simulink model "Master_Slave_No_Force_Control"  (R2020a)
settings: Solver=VariableStepAuto  StartTime=0.0  StopTime=1000  RelTol=1e-3
values from neighbouring files (symbols this model uses):
  B = 100    [Teleop_parameters.m]    (also in base.mat = 0.0517063081696; base_no_attrito.mat = 0; ci_siamo.mat = 0.0517063081696; force_control.mat = 0.0517063081696)
  Be = 10^3    (= 1000)    [Teleop_parameters.m]    (also in base.mat = 0.5; base_no_attrito.mat = 0.5; ci_siamo.mat = 5; force_control.mat = 0.5)
  Bh = 0.02    [Teleop_parameters.m]    (also in base.mat; base_no_attrito.mat; ci_siamo.mat; force_control.mat)
  Bl = 0.02    [Teleop_parameters.m]
  Fc_h = 5    [Teleop_parameters.m]    (also in base.mat; base_no_attrito.mat; ci_siamo.mat; force_control.mat)
  J = 50    [Teleop_parameters.m]    (also in base.mat = 0.0629265770424; base_no_attrito.mat = 0.0629265770424; ci_siamo.mat = 0.0629265770424; force_control.mat = 0.0629265770424)
  Jh = 0.02    [Teleop_parameters.m]    (also in base.mat; base_no_attrito.mat; ci_siamo.mat; force_control.mat)
  Jl = 0.03    [Teleop_parameters.m]
  Kc2v_m = 2    [Teleop_parameters.m]    (also in base.mat; base_no_attrito.mat; ci_siamo.mat; force_control.mat)
  Kc2v_s = 2    [Teleop_parameters.m]    (also in base.mat; base_no_attrito.mat; ci_siamo.mat; force_control.mat)
  Kd_h = 0.5    [Teleop_parameters.m]    (also in base.mat = 1; base_no_attrito.mat = 1; ci_siamo.mat = 10; force_control.mat = 1)
  Kd_m = 6    [Teleop_parameters.m]    (also in base.mat = 1; base_no_attrito.mat = 1; ci_siamo.mat = 0.005; force_control.mat = 1)
  Kd_s = 6    [Teleop_parameters.m]    (also in base.mat = 1; base_no_attrito.mat = 1; ci_siamo.mat = 0.5; force_control.mat = 1)
  Ke = 2    [Teleop_parameters.m]    (also in base.mat = 10; base_no_attrito.mat = 10; ci_siamo.mat = 10; force_control.mat = 10)
  Km = 2    [Teleop_parameters.m]
  Kp_h = 1.2    [Teleop_parameters.m]    (also in base.mat; base_no_attrito.mat; ci_siamo.mat = 10; force_control.mat)
  Kp_m = 200    [Teleop_parameters.m]    (also in base.mat = 1; base_no_attrito.mat = 1; ci_siamo.mat = 0.01; force_control.mat = 1)
  Kp_s = 200    [Teleop_parameters.m]    (also in base.mat = 1; base_no_attrito.mat = 1; ci_siamo.mat = 1; force_control.mat = 1)
  Kt2c_m = 1.182    [Teleop_parameters.m]    (also in base.mat; base_no_attrito.mat; ci_siamo.mat; force_control.mat)
  Kt2c_s = 1.182    [Teleop_parameters.m]    (also in base.mat; base_no_attrito.mat; ci_siamo.mat; force_control.mat)
  L = 0.0025    [Teleop_parameters.m]
  lArm_m = 0.1    [Teleop_parameters.m]    (also in base.mat; base_no_attrito.mat; ci_siamo.mat; force_control.mat)
  lArm_s = 0.1    [Teleop_parameters.m]    (also in base.mat; base_no_attrito.mat; ci_siamo.mat; force_control.mat)
  maxCurrent_m = 4.5    [Teleop_parameters.m]    (also in base.mat; base_no_attrito.mat; ci_siamo.mat; force_control.mat)
  maxCurrent_s = 4.5    [Teleop_parameters.m]    (also in base.mat; base_no_attrito.mat; ci_siamo.mat; force_control.mat)
  N = 1    [Teleop_parameters.m]
  qe = 1    [Teleop_parameters.m]    (also in base.mat = 5; base_no_attrito.mat = 5; ci_siamo.mat = 0.5; force_control.mat = 5)
  R = 0.434    [Teleop_parameters.m]
settings Model: Creator=kriato  LastModifiedBy=giovanni

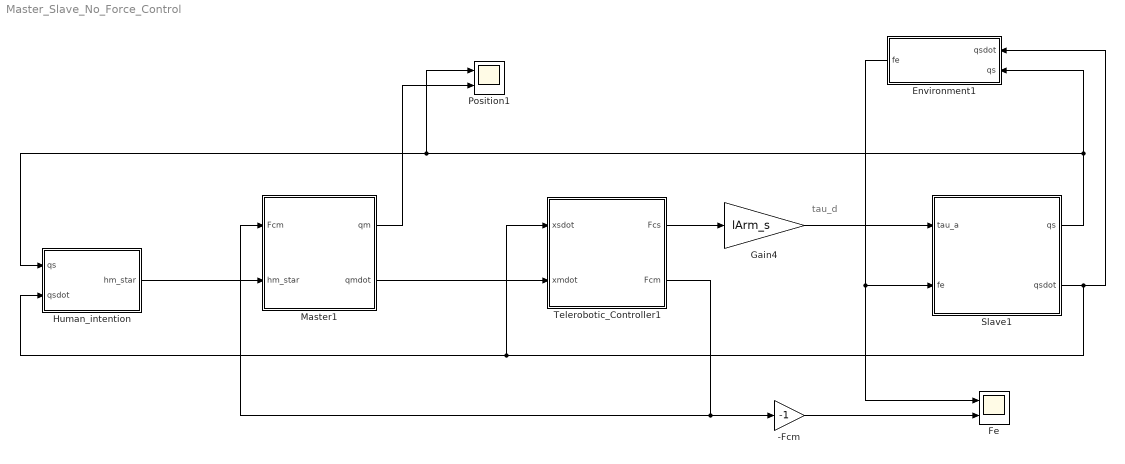
== system Master_Slave_No_Force_Control ==
  note: tau_d
  -Fcm : Gain  Gain=-1
  Environment1 : Subsystem
  Fe : Scope  NumInputPorts=2
  Gain4 : Gain  Gain=lArm_s
  Human_intention : Subsystem
  Master1 : Subsystem
  Position1 : Scope  NumInputPorts=2
  Slave1 : Subsystem
  Telerobotic_Controller1 : Subsystem
  wires:
  Gain4/1 -> Slave1/1(tau_a)
  Master1/1(qm) -> Position1/2
  Environment1/1(fe) -> Fe/1, Slave1/2(fe)
  Telerobotic_Controller1/1(Fcs) -> Gain4/1
  Slave1/1(qs) -> Environment1/2(qs), Human_intention/1(qs), Position1/1
  Telerobotic_Controller1/2(Fcm) -> Master1/1(Fcm), -Fcm/1
  -Fcm/1 -> Fe/2
  Slave1/2(qsdot) -> Human_intention/2(qsdot), Telerobotic_Controller1/1(xsdot), Environment1/1(qsdot)
  Human_intention/1(hm_star) -> Master1/2(hm_star)
  Master1/2(qmdot) -> Telerobotic_Controller1/2(xmdot)

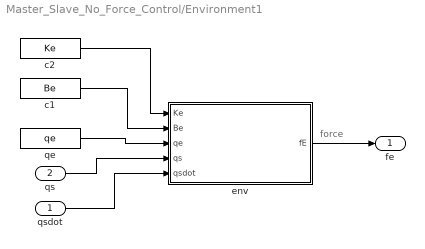
== system Master_Slave_No_Force_Control/Environment1 ==
  note: force
  qsdot : Inport
  qs : Inport  Port=2
  c1 : Constant  Value=Be  SampleTime=0
  c2 : Constant  Value=Ke  SampleTime=0
  env : MATLAB Function  TreatAsAtomicUnit=on
  qe : Constant  Value=qe  SampleTime=0
  fe : Outport  VectorParamsAs1DForOutWhenUnconnected=off
  wires:
  qe/1 -> env/3(qe)
  c1/1 -> env/2(Be)
  c2/1 -> env/1(Ke)
  qs/1 -> env/4(qs)
  qsdot/1 -> env/5(qsdot)
  env/1(fE) -> fe/1

== system Master_Slave_No_Force_Control/Human_intention ==
  qs : Inport
  qsdot : Inport  Port=2
  Operator (intention) : Subsystem
  Subsystem : Subsystem
  hm_star : Outport
  wires:
  Subsystem/1(qm_ref) -> Operator (intention)/3(qm_ref)
  Subsystem/2(qmdot_ref) -> Operator (intention)/4(qmdot_ref)
  Operator (intention)/1(hm_star) -> hm_star/1
  qs/1 -> Operator (intention)/1(qs)
  qsdot/1 -> Operator (intention)/2(qsdot)

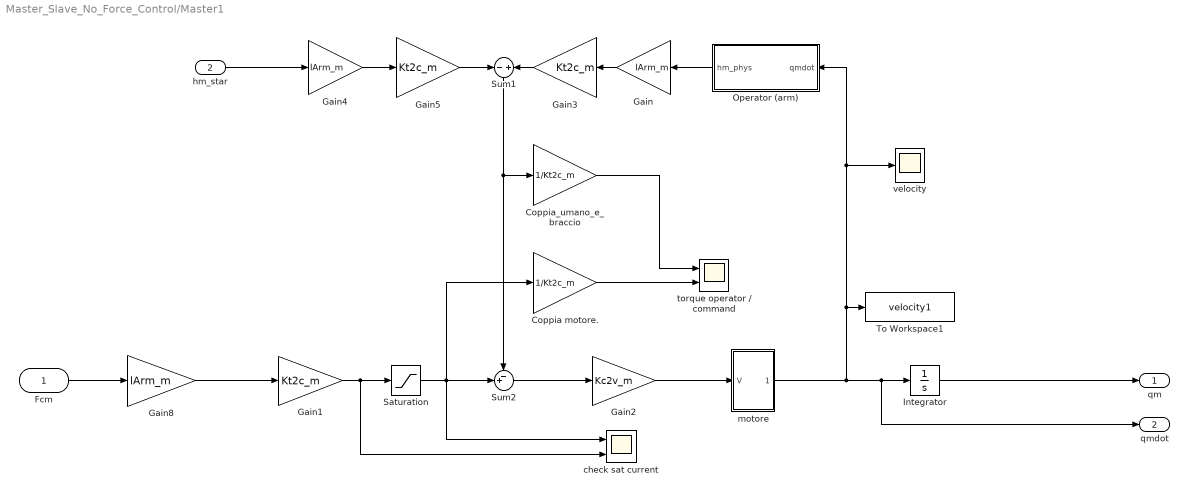
== system Master_Slave_No_Force_Control/Master1 ==
  Fcm : Inport
  hm_star : Inport  Port=2
  Coppia motore. : Gain  Gain=1/Kt2c_m
  Coppia_umano_e_braccio : Gain  Gain=1/Kt2c_m
  Gain : Gain  Gain=lArm_m
  Gain1 : Gain  Gain=Kt2c_m
  Gain2 : Gain  Gain=Kc2v_m
  Gain3 : Gain  Gain=Kt2c_m
  Gain4 : Gain  Gain=lArm_m
  Gain5 : Gain  Gain=Kt2c_m
  Gain8 : Gain  Gain=lArm_m
  Integrator : Integrator
  Operator (arm) : Subsystem
  Saturation : Saturate  UpperLimit=maxCurrent_m  LowerLimit=-maxCurrent_m
  Sum1 : Sum  Inputs=-+
  Sum2 : Sum  Inputs=-+|
  To Workspace1 : ToWorkspace  VariableName=velocity1  SaveFormat=Timeseries  SampleTime=-1
  check sat current : Scope  NumInputPorts=2
  motore : Subsystem
  torque operator / command : Scope  NumInputPorts=2
  velocity : Scope
  qm : Outport
  qmdot : Outport  Port=2
  wires:
  Integrator/1 -> qm/1
  Sum2/1 -> Gain2/1
  Gain3/1 -> Sum1/2
  Gain2/1 -> motore/1(V)
  Gain1/1 -> check sat current/2, Saturation/1
  Coppia_umano_e_braccio/1 -> torque operator / command/1
  Coppia motore./1 -> torque operator / command/2
  motore/1(qdot) -> velocity/1, Operator (arm)/1(qmdot), To Workspace1/1, qmdot/1, Integrator/1
  Gain8/1 -> Gain1/1
  Gain5/1 -> Sum1/1
  Operator (arm)/1(hm_phys) -> Gain/1
  Sum1/1 -> Sum2/1, Coppia_umano_e_braccio/1
  Saturation/1 -> Coppia motore./1, Sum2/2, check sat current/1
  Gain/1 -> Gain3/1
  Gain4/1 -> Gain5/1
  Fcm/1 -> Gain8/1
  hm_star/1 -> Gain4/1

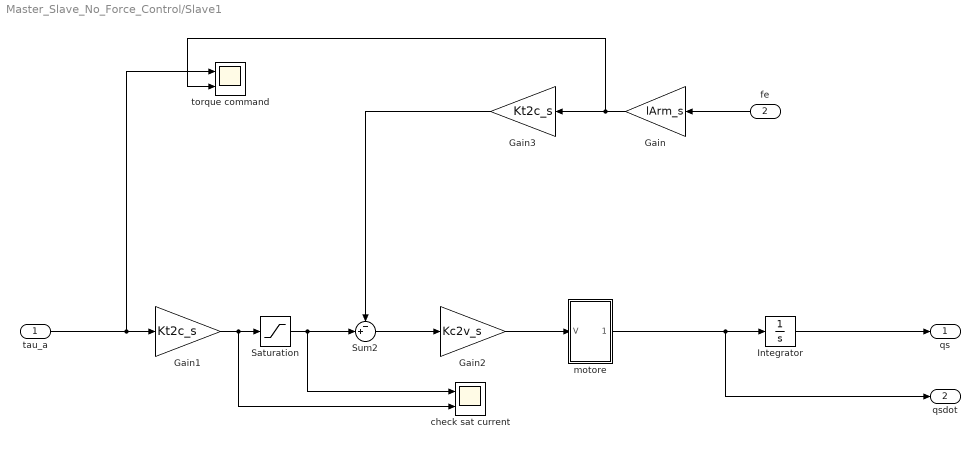
== system Master_Slave_No_Force_Control/Slave1 ==
  tau_a : Inport
  fe : Inport  Port=2
  Gain : Gain  Gain=lArm_s
  Gain1 : Gain  Gain=Kt2c_s
  Gain2 : Gain  Gain=Kc2v_s
  Gain3 : Gain  Gain=Kt2c_s
  Integrator : Integrator
  Saturation : Saturate  UpperLimit=maxCurrent_s  LowerLimit=-maxCurrent_s
  Sum2 : Sum  Inputs=-+|
  check sat current : Scope  NumInputPorts=2
  motore : Subsystem
  torque command : Scope  NumInputPorts=2
  qs : Outport
  qsdot : Outport  Port=2
  wires:
  Integrator/1 -> qs/1
  Sum2/1 -> Gain2/1
  Saturation/1 -> Sum2/2, check sat current/1
  Gain2/1 -> motore/1(V)
  motore/1(qdot) -> qsdot/1, Integrator/1
  Gain1/1 -> check sat current/2, Saturation/1
  tau_a/1 -> torque command/1, Gain1/1
  Gain3/1 -> Sum2/1
  fe/1 -> Gain/1
  Gain/1 -> Gain3/1, torque command/2

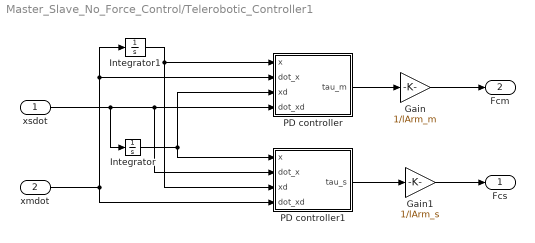
== system Master_Slave_No_Force_Control/Telerobotic_Controller1 ==
  xsdot : Inport
  xmdot : Inport  Port=2
  Gain : Gain  Gain=1/lArm_m
  Gain1 : Gain  Gain=1/lArm_s
  Integrator : Integrator
  Integrator1 : Integrator
  PD controller : Subsystem
  PD controller1 : Subsystem
  Fcs : Outport
  Fcm : Outport  Port=2
  wires:
  Integrator/1 -> PD controller1/1(x), PD controller/3(xd)
  Integrator1/1 -> PD controller1/3(xd), PD controller/1(x)
  xsdot/1 -> PD controller1/2(dot_x), PD controller/4(dot_xd), Integrator/1
  PD controller1/1(tau_s) -> Gain1/1
  PD controller/1(tau_m) -> Gain/1
  xmdot/1 -> PD controller1/4(dot_xd), PD controller/2(dot_x), Integrator1/1
  Gain/1 -> Fcm/1
  Gain1/1 -> Fcs/1

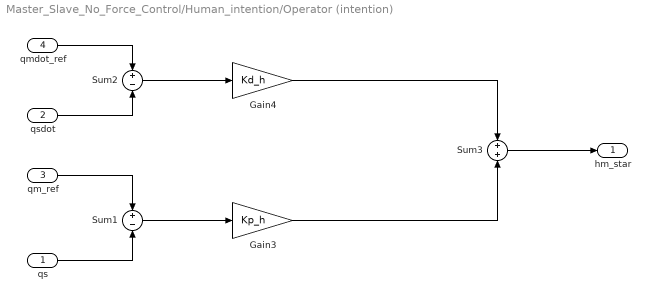
== system Master_Slave_No_Force_Control/Human_intention/Operator (intention) ==
  qs : Inport
  qsdot : Inport  Port=2
  qm_ref : Inport  Port=3
  qmdot_ref : Inport  Port=4
  Gain3 : Gain  Gain=Kp_h
  Gain4 : Gain  Gain=Kd_h
  Sum1 : Sum  Inputs=+|-
  Sum2 : Sum  Inputs=+|-
  Sum3 : Sum  Inputs=+|+
  hm_star : Outport  VectorParamsAs1DForOutWhenUnconnected=off
  wires:
  qs/1 -> Sum1/2
  qm_ref/1 -> Sum1/1
  qmdot_ref/1 -> Sum2/1
  Sum1/1 -> Gain3/1
  qsdot/1 -> Sum2/2
  Sum2/1 -> Gain4/1
  Gain4/1 -> Sum3/1
  Gain3/1 -> Sum3/2
  Sum3/1 -> hm_star/1

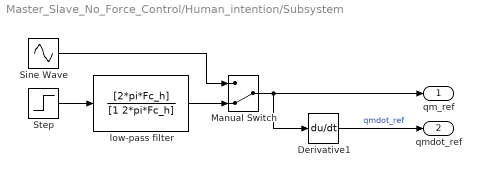
== system Master_Slave_No_Force_Control/Human_intention/Subsystem ==
  Derivative1 : Derivative  CoefficientInTFapproximation=0.001
  Manual Switch : ManualSwitch  CurrentSetting=0
  Sine Wave : Sin  SampleTime=0
  Step : Step  SampleTime=0
  low-pass filter : TransferFcn  Numerator=[2*pi*Fc_h]  Denominator=[1 2*pi*Fc_h]
  qm_ref : Outport
  qmdot_ref : Outport  Port=2
  wires:
  low-pass filter/1 -> Manual Switch/2
  Manual Switch/1 -> qm_ref/1, Derivative1/1
  Derivative1/1 -> qmdot_ref/1  "qmdot_ref"
  Step/1 -> low-pass filter/1
  Sine Wave/1 -> Manual Switch/1

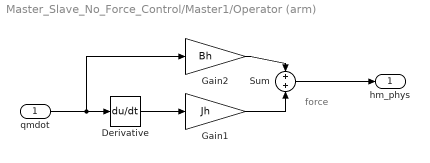
== system Master_Slave_No_Force_Control/Master1/Operator (arm) ==
  note: force
  qmdot : Inport
  Derivative : Derivative  CoefficientInTFapproximation=0.001
  Gain1 : Gain  Gain=Jh
  Gain2 : Gain  Gain=Bh
  Sum : Sum  Inputs=+|+
  hm_phys : Outport  VectorParamsAs1DForOutWhenUnconnected=off
  wires:
  qmdot/1 -> Gain2/1, Derivative/1
  Sum/1 -> hm_phys/1
  Derivative/1 -> Gain1/1
  Gain2/1 -> Sum/1
  Gain1/1 -> Sum/2

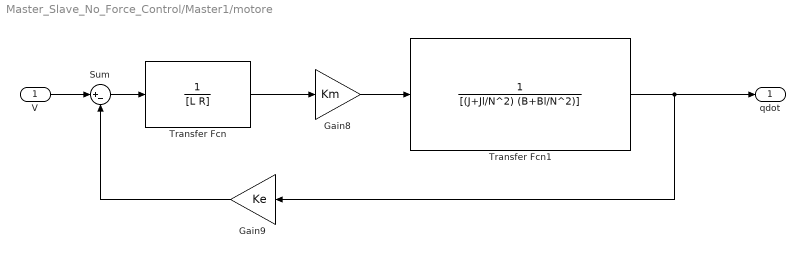
== system Master_Slave_No_Force_Control/Master1/motore ==
  V : Inport
  Gain8 : Gain  Gain=Km
  Gain9 : Gain  Gain=Ke
  Sum : Sum  Inputs=|+-
  Transfer Fcn : TransferFcn  Denominator=[L R]
  Transfer Fcn1 : TransferFcn  Denominator=[(J+Jl/N^2) (B+Bl/N^2)]
  qdot : Outport
  wires:
  Sum/1 -> Transfer Fcn/1
  V/1 -> Sum/1
  Transfer Fcn/1 -> Gain8/1
  Gain9/1 -> Sum/2
  Gain8/1 -> Transfer Fcn1/1
  Transfer Fcn1/1 -> Gain9/1, qdot/1

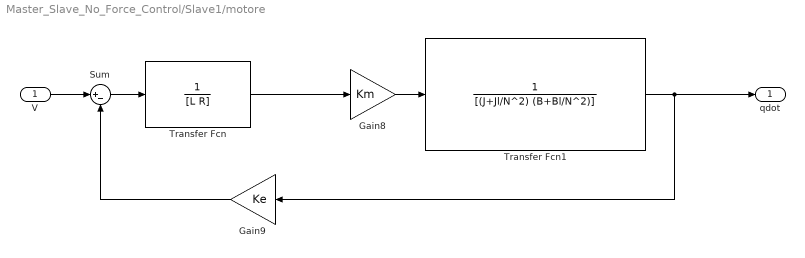
== system Master_Slave_No_Force_Control/Slave1/motore ==
  V : Inport
  Gain8 : Gain  Gain=Km
  Gain9 : Gain  Gain=Ke
  Sum : Sum  Inputs=|+-
  Transfer Fcn : TransferFcn  Denominator=[L R]
  Transfer Fcn1 : TransferFcn  Denominator=[(J+Jl/N^2) (B+Bl/N^2)]
  qdot : Outport
  wires:
  Sum/1 -> Transfer Fcn/1
  V/1 -> Sum/1
  Transfer Fcn/1 -> Gain8/1
  Gain9/1 -> Sum/2
  Gain8/1 -> Transfer Fcn1/1
  Transfer Fcn1/1 -> Gain9/1, qdot/1

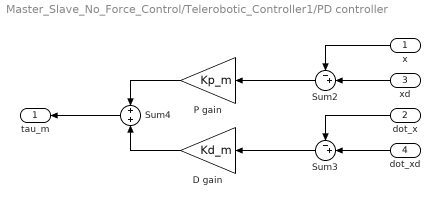
== system Master_Slave_No_Force_Control/Telerobotic_Controller1/PD controller ==
  x : Inport
  dot_x : Inport  Port=2
  xd : Inport  Port=3
  dot_xd : Inport  Port=4
  D gain : Gain  Gain=Kd_m
  P gain : Gain  Gain=Kp_m
  Sum2 : Sum  Inputs=-+|
  Sum3 : Sum  Inputs=-+|
  Sum4 : Sum
  tau_m : Outport  VectorParamsAs1DForOutWhenUnconnected=off
  wires:
  D gain/1 -> Sum4/2
  dot_x/1 -> Sum3/1
  dot_xd/1 -> Sum3/2
  x/1 -> Sum2/1
  xd/1 -> Sum2/2
  Sum3/1 -> D gain/1
  P gain/1 -> Sum4/1
  Sum4/1 -> tau_m/1
  Sum2/1 -> P gain/1

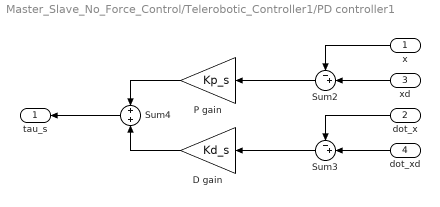
== system Master_Slave_No_Force_Control/Telerobotic_Controller1/PD controller1 ==
  x : Inport
  dot_x : Inport  Port=2
  xd : Inport  Port=3
  dot_xd : Inport  Port=4
  D gain : Gain  Gain=Kd_s
  P gain : Gain  Gain=Kp_s
  Sum2 : Sum  Inputs=-+|
  Sum3 : Sum  Inputs=-+|
  Sum4 : Sum
  tau_s : Outport  VectorParamsAs1DForOutWhenUnconnected=off
  wires:
  D gain/1 -> Sum4/2
  dot_x/1 -> Sum3/1
  dot_xd/1 -> Sum3/2
  x/1 -> Sum2/1
  xd/1 -> Sum2/2
  Sum3/1 -> D gain/1
  P gain/1 -> Sum4/1
  Sum4/1 -> tau_s/1
  Sum2/1 -> P gain/1

== matlab function Master_Slave_No_Force_Control/Environment1/env ==
  data: Ke input; Be input; qe input; qs input; fE output; qsdot input
function fE  = environment(Ke, Be, qe, qs, qsdot)
if qs > qe
   fE = Ke * (qs - qe) + Be * qsdot;
else
   fE = 0;
end
